simulink model "ideal_Highpass_Lowpass_Pair"  (R2014b)
settings: Solver=ode45  StartTime=0.0  StopTime=5  RelTol=1e-3
settings Model: Creator=brownaa  LastModifiedBy=brownaa

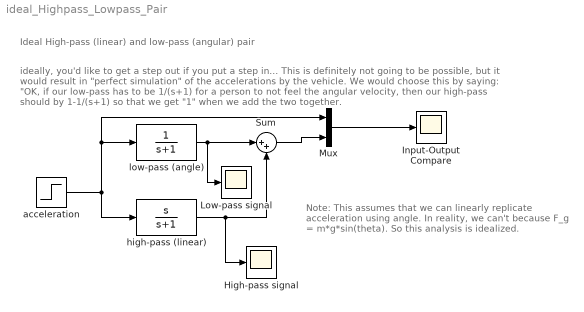
== system ideal_Highpass_Lowpass_Pair ==
  note: Note: This assumes that we can linearly replicate
      | acceleration using angle. In reality, we can't because
      | F_g = m*g*sin(theta). So this analysis is idealized.
  note: ideally, you'd like to get a step out if you put a step in... This is definitely not going to be possible,
      | but it would result in "perfect simulation" of the accelerations by the vehicle. We would choose this by saying: "OK, if our low-pass has to be 1/(s+1) for a person to not feel the angular velocity, then our high-pass should by 1-1/(s+1) so that we get "1" when we add the two together.
  note: Ideal High-pass (linear) and low-pass (angular) pair
  High-pass signal : Scope
  Input-Output Compare : Scope
  Low-pass signal : Scope
      settings: SaveName=ScopeData2
  Mux : Mux  Inputs=2
  Sum : Sum  Inputs=|++
  acceleration : Step  SampleTime=0
  high-pass (linear) : TransferFcn  Numerator=[1 0]  Denominator=[1 1]
  low-pass (angle) : TransferFcn  Denominator=[1 1]
  wires:
  acceleration/1 -> high-pass (linear)/1, Mux/1, low-pass (angle)/1
  low-pass (angle)/1 -> Low-pass signal/1, Sum/1
  high-pass (linear)/1 -> High-pass signal/1, Sum/2
  Sum/1 -> Mux/2
  Mux/1 -> Input-Output Compare/1
